simulink model "project_3"  (R2019a)
settings: Solver=VariableStepAuto  StartTime=0.0  StopTime=Sim_Time  MaxStep=0.01  RelTol=1e-3
values from neighbouring files (symbols this model uses):
  b = 3.5077E-6    (= 3.5077e-06)    [project_10_run.m]    (also in project_3.m = 0.3; project_4_run.m = 0.1; project_7_run.m = 10; project_8_run.m = 10)
  k = 10    [project_3.m]    (also in project_4_run.m = 20; project_7_run.m = 20; project_8_run.m = 20)
  M = 1    [project_3.m]    (also in project_4_run.m; project_7_run.m; project_8_run.m)
settings Model: Creator=Nikita  LastModifiedBy=Nikita

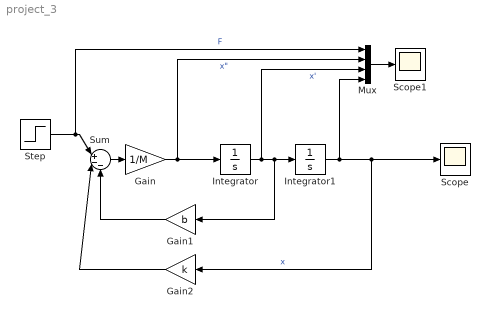
== system project_3 ==
  Gain : Gain  Gain=1/M
  Gain1 : Gain  Gain=b
  Gain2 : Gain  Gain=k
  Integrator : Integrator
  Integrator1 : Integrator
  Mux : Mux
  Scope : Scope
  Scope1 : Scope
  Step : Step  After=M  SampleTime=0
  Sum : Sum  Inputs=|+--
  wires:
  Sum/1 -> Gain/1
  Gain/1 -> Mux/2, Integrator/1  "x\""
  Integrator/1 -> Mux/3, Integrator1/1, Gain1/1  "x'"
  Integrator1/1 -> Mux/4, Gain2/1, Scope/1  "x"
  Gain1/1 -> Sum/3
  Gain2/1 -> Sum/2
  Step/1 -> Mux/1, Sum/1  "F"
  Mux/1 -> Scope1/1
